simulink model "block_diagram"  (Simulink 6.3)
settings: Solver=ode3  StartTime=0.0  StopTime=10.0  FixedStep=0.0001  RelTol=1e-3
values from neighbouring files (symbols this model uses):
  b_1 = 0    [parameters.m]
  b_op = damping_vec(b)    [automated_bode.m]    (also in find_tf.m = 1000000000; parameters.m = 100; parameters2.m = 20)
  b_spring = spring_damping_vec(b_sp)    [automated_bode.m]    (also in parameters.m = 0.01; parameters2.m = 100)
  dx_max = dist_min - dist_max    (= -0.0018)    [parameters.m]    (also in parameters2.m)
  freq = frequency_vec(i)    [automated_bode.m]    (also in parameters.m = 100; parameters2.m = 1)
  J_T = 1.25E-3 / n / n    (= 9.96492346939e-08)    [analytical_bode_comparing.m]    (also in analytical_bode_creator.m; find_tf.m; parameters.m; parameters2.m)
  K_ampl = 10    [analytical_bode_comparing.m]    (also in parameters.m; parameters2.m)
  K_emf = 3.29E-3 / 60    (= 5.48333333333e-05)    [analytical_bode_comparing.m]    (also in analytical_bode_creator.m; find_tf.m; parameters.m; parameters2.m)
  k_eq = spring_stiffness_vec(k)    [analytical_bode_comparing.m]    (also in analytical_bode_creator.m = 6; find_tf.m = 6; parameters.m = 6000; parameters2.m = 6000)
  k_op = stiffness_vec(k)    [automated_bode.m]    (also in find_tf.m = 1000000000; parameters.m = 100; parameters2.m = 200)
  K_tau = efficiency*31.4E-3    (= 0.01884)    [analytical_bode_comparing.m]    (also in analytical_bode_creator.m = 0.0314; find_tf.m = 0.0314; parameters.m = 0.0314; parameters2.m = 0.0314)
  K_Vto8bit = 51    [parameters.m]
  L_a = 5.8E-3    (= 0.0058)    [analytical_bode_comparing.m]    (also in analytical_bode_creator.m; find_tf.m; parameters.m; parameters2.m)
  L_CL = 20E-3    (= 0.02)    [analytical_bode_comparing.m]    (also in analytical_bode_creator.m; calc_JTOT.m; find_tf.m; parameters.m)
  limit_val = 2 * MOTOR_MAX_V * K_Vto8bit / K_ampl    (= 204)    [parameters.m]
  m_2 = 7E-3    (= 0.007)    [analytical_bode_comparing.m]    (also in analytical_bode_creator.m; find_tf.m; parameters.m; parameters2.m)
  n = 112    [analytical_bode_comparing.m]    (also in analytical_bode_creator.m; calc_JTOT.m; find_tf.m; parameters.m)
  R_a = 118.6    [analytical_bode_comparing.m]    (also in analytical_bode_creator.m; find_tf.m; parameters.m; parameters2.m)
  V_offset = -20    [parameters.m]    (also in parameters2.m = -25)
libraries: simulink_extras x1
settings Model: LastModifiedBy=oechslin

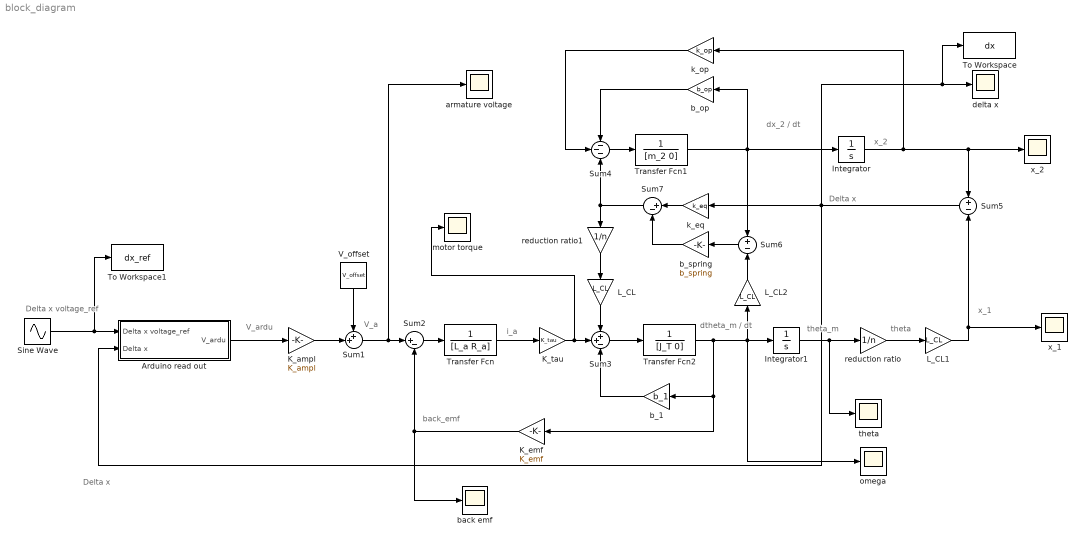
== system block_diagram ==
  note: Delta x voltage_ref
  note: x_2
  note: Delta x
  note: x_1
  note: dtheta_m / dt
  note: theta_m
  note: back_emf
  note: V_a
  note: V_ardu
  note: Delta x
  note: theta
  note: dx_2 / dt
  note: i_a
  Arduino read out : Subsystem
  Integrator : Integrator
  Integrator1 : Integrator
  K_ampl : Gain  Gain=K_ampl
  K_emf : Gain  Orientation=left  Gain=K_emf
  K_tau : Gain  Gain=K_tau
  L_CL : Gain  Orientation=down  Gain=L_CL
  L_CL1 : Gain  Gain=L_CL
  L_CL2 : Gain  Orientation=up  Gain=L_CL
  Sine Wave : Sin  Amplitude=2  Bias=2.5  Frequency=freq * 2*3.1416  SampleTime=0
  Sum1 : Sum  Inputs=++|
  Sum2 : Sum  Inputs=|+-
  Sum3 : Sum  Inputs=++-
  Sum4 : Sum  Inputs=---
  Sum5 : Sum  Orientation=left  Inputs=+|-
  Sum6 : Sum  Orientation=left  Inputs=+|-
  Sum7 : Sum  Orientation=left  Inputs=|+-
  To Workspace : ToWorkspace  VariableName=dx  SampleTime=-1  SaveFormat=Structure
  To Workspace1 : ToWorkspace  VariableName=dx_ref  SampleTime=-1  SaveFormat=Structure
  Transfer Fcn : TransferFcn  Denominator=[L_a R_a]
  Transfer Fcn1 : TransferFcn  Denominator=[m_2 0]
  Transfer Fcn2 : TransferFcn  Denominator=[J_T 0]
  V_offset : Constant  Orientation=down  Value=V_offset
  armature voltage : Scope
      settings: TimeRange=10
  b_1 : Gain  Orientation=left  Gain=b_1
  b_op : Gain  Orientation=left  Gain=b_op
  b_spring : Gain  Orientation=left  Gain=b_spring
  back emf : Scope
      settings: TimeRange=10  SaveName=ScopeData6
  delta x : Scope
      settings: TimeRange=10
  k_eq : Gain  Orientation=left  Gain=k_eq
  k_op : Gain  Orientation=left  Gain=k_op
  motor torque : Scope
      settings: TimeRange=10  SaveName=ScopeData3
  omega : Scope
      settings: TimeRange=10  SaveName=ScopeData4
  reduction ratio : Gain  Gain=1/n
  reduction ratio1 : Gain  Orientation=down  Gain=1/n
  theta : Scope
      settings: TimeRange=10  SaveName=ScopeData7
  x_1 : Scope
      settings: TimeRange=10  SaveName=ScopeData8
  x_2 : Scope
      settings: TimeRange=10  SaveName=ScopeData5
  wires:
  V_offset/1 -> Sum1/1
  K_ampl/1 -> Sum1/2
  Arduino read out/1(V_ardu) -> K_ampl/1
  Sum1/1 -> Sum2/1, armature voltage/1
  Sum2/1 -> Transfer Fcn/1
  Transfer Fcn/1 -> K_tau/1
  L_CL/1 -> Sum3/1
  K_tau/1 -> Sum3/2, motor torque/1
  Sum4/1 -> Transfer Fcn1/1
  b_op/1 -> Sum4/1
  Integrator/1 -> k_op/1, Sum5/1, x_2/1
  Sum5/1 -> k_eq/1, Arduino read out/2(Delta x), delta x/1, To Workspace/1
  L_CL1/1 -> Sum5/2, x_1/1
  Integrator1/1 -> reduction ratio/1, theta/1
  Transfer Fcn2/1 -> b_1/1, K_emf/1, Integrator1/1, omega/1, L_CL2/1
  Sum3/1 -> Transfer Fcn2/1
  b_1/1 -> Sum3/3
  K_emf/1 -> Sum2/2, back emf/1
  Sine Wave/1 -> Arduino read out/1(Delta x voltage_ref), To Workspace1/1
  reduction ratio/1 -> L_CL1/1
  reduction ratio1/1 -> L_CL/1
  k_op/1 -> Sum4/2
  L_CL2/1 -> Sum6/2
  Sum6/1 -> b_spring/1
  b_spring/1 -> Sum7/2
  k_eq/1 -> Sum7/1
  Sum7/1 -> reduction ratio1/1, Sum4/3
  Transfer Fcn1/1 -> Integrator/1, Sum6/1, b_op/1

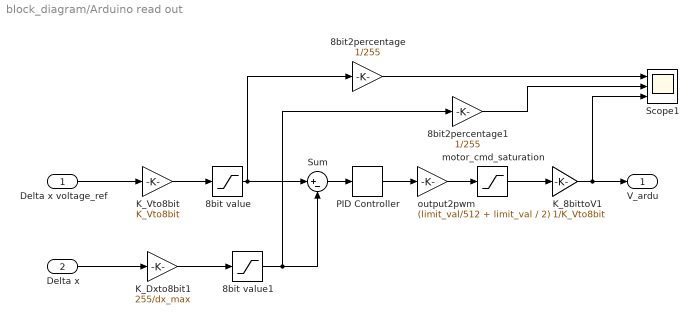
== system block_diagram/Arduino read out ==
  Delta x voltage_ref : Inport
  Delta x : Inport  Port=2
  8bit value : Saturate  UpperLimit=255  LowerLimit=0
  8bit value1 : Saturate  UpperLimit=255  LowerLimit=0
  8bit2percentage : Gain  Gain=1/255
  8bit2percentage1 : Gain  Gain=1/255
  K_8bittoV1 : Gain  Gain=1/K_Vto8bit
  K_Dxto8bit1 : Gain  Gain=255/dx_max
  K_Vto8bit : Gain  Gain=K_Vto8bit
  PID Controller : simulink_extras/Additional Linear/PID Controller  P=1  I=0  D=0
  Scope1 : Scope  NumInputPorts=3
      settings: TimeRange=10  YMin=-5~-5~-5  YMax=5~5~5  SaveName=ScopeData2
  Sum : Sum  Inputs=|+-
  motor_cmd_saturation : Saturate  UpperLimit=limit_val  LowerLimit=0
  output2pwm : Gain  Gain=(limit_val/512 + limit_val / 2)
  V_ardu : Outport
  wires:
  Delta x voltage_ref/1 -> K_Vto8bit/1
  Delta x/1 -> K_Dxto8bit1/1
  Sum/1 -> PID Controller/1
  PID Controller/1 -> output2pwm/1
  output2pwm/1 -> motor_cmd_saturation/1
  K_Dxto8bit1/1 -> 8bit value1/1
  8bit value1/1 -> Sum/2, 8bit2percentage1/1
  K_Vto8bit/1 -> 8bit value/1
  8bit value/1 -> Sum/1, 8bit2percentage/1
  motor_cmd_saturation/1 -> K_8bittoV1/1
  8bit2percentage/1 -> Scope1/1
  8bit2percentage1/1 -> Scope1/2
  K_8bittoV1/1 -> V_ardu/1, Scope1/3
